simulink model "pwm_controlled_system"  (R2017a)
settings: Solver=FixedStepAuto  StartTime=0.0  StopTime=t_f  FixedStep=1e-6  RelTol=1e-3
values from neighbouring files (symbols this model uses):
  A = double(subs(A_sym, symbs, vals))    [load_params.m]
  B = double(subs(B_sym, symbs, vals))    [load_params.m]
  C = double(subs(C_sym, symbs, vals))    [load_params.m]    (also in load_pwm_avg_pred_controller.m = sysd.c; load_pwm_pred_controller.m = sysd.c)
  Ctilde = double(subs(Ctilde_sym, symbs, vals))    [load_params.m]
  torque_ref = n_val*k_i_val*i_ref    [load_params.m]
  Tpwm_val = 1e-2    (= 0.01)    [load_params.m]    (also in ss_value.m = 0.001)
  Ts_val = 1e-1    (= 0.1)    [load_params.m]    (also in ss_value.m = 0.011)
  Vcc_val = 12    [load_params.m]
  x0 = [0; 0]    [sim_controlled_system.m]
settings Model: Creator=brunolnetto  LastModifiedBy=brunolnetto

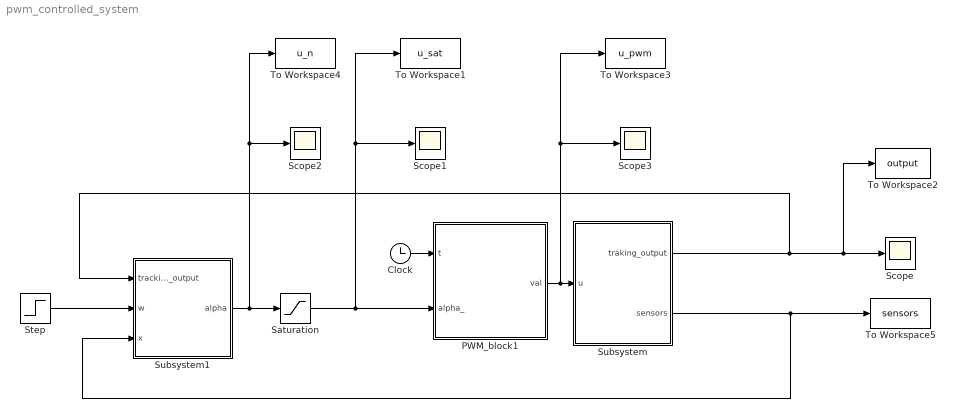
== system pwm_controlled_system ==
  Clock : Clock
  PWM_block1 : MATLAB Function  TreatAsAtomicUnit=on
  Saturation : Saturate  UpperLimit=1  LowerLimit=-1
  Scope{,1..3} (4 alike) : Scope
  Step : Step  Time=0  After=torque_ref  SampleTime=Ts_val
  Subsystem : Subsystem
  Subsystem1 : Subsystem
  To Workspace1 : ToWorkspace  VariableName=u_sat  SaveFormat=Structure With Time  SampleTime=-1
  To Workspace2 : ToWorkspace  VariableName=output  SaveFormat=Structure With Time  SampleTime=-1
  To Workspace3 : ToWorkspace  VariableName=u_pwm  SaveFormat=Structure With Time  SampleTime=-1
  To Workspace4 : ToWorkspace  VariableName=u_n  SaveFormat=Structure With Time  SampleTime=-1
  To Workspace5 : ToWorkspace  VariableName=sensors  SaveFormat=Structure With Time  SampleTime=-1
  wires:
  Subsystem/1(traking_output) -> To Workspace2/1, Scope/1, Subsystem1/1(tracking_output)
  Subsystem/2(sensors) -> To Workspace5/1, Subsystem1/3(x)
  Step/1 -> Subsystem1/2(w)
  Clock/1 -> PWM_block1/1(t)
  Subsystem1/1(alpha) -> To Workspace4/1, Scope2/1, Saturation/1
  Saturation/1 -> PWM_block1/2(alpha_), Scope1/1, To Workspace1/1
  PWM_block1/1(val) -> Scope3/1, To Workspace3/1, Subsystem/1(u)

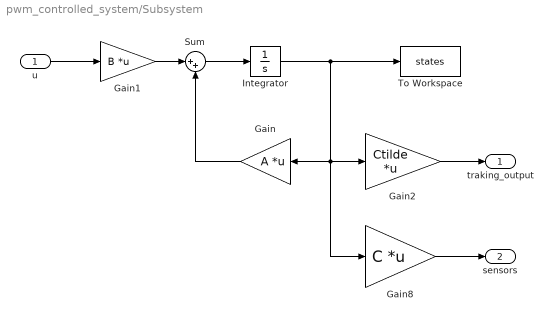
== system pwm_controlled_system/Subsystem ==
  u : Inport
  Gain : Gain  Gain=A  Multiplication=Matrix(K*u) (u vector)
  Gain1 : Gain  Gain=B  Multiplication=Matrix(K*u) (u vector)
  Gain2 : Gain  Gain=Ctilde  Multiplication=Matrix(K*u) (u vector)
  Gain8 : Gain  Gain=C  Multiplication=Matrix(K*u) (u vector)
  Integrator : Integrator  InitialCondition=x0
  Sum : Sum  Inputs=|++
  To Workspace : ToWorkspace  VariableName=states  SaveFormat=Structure With Time  SampleTime=-1
  traking_output : Outport
  sensors : Outport  Port=2
  wires:
  Gain8/1 -> sensors/1
  Gain1/1 -> Sum/1
  Integrator/1 -> To Workspace/1, Gain2/1, Gain8/1, Gain/1
  u/1 -> Gain1/1
  Gain/1 -> Sum/2
  Sum/1 -> Integrator/1
  Gain2/1 -> traking_output/1

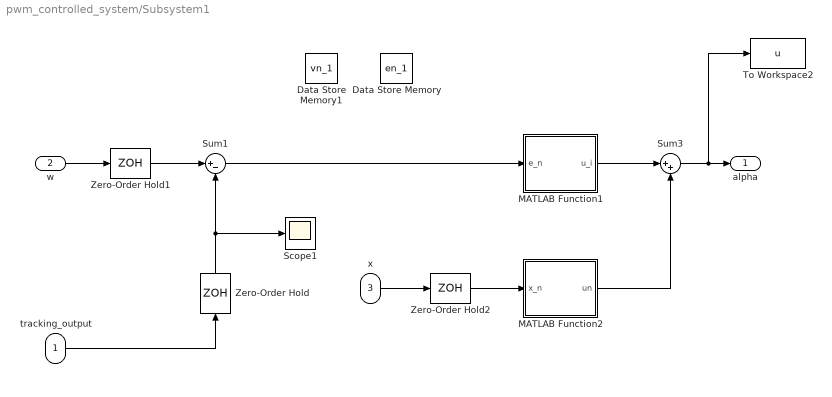
== system pwm_controlled_system/Subsystem1 ==
  tracking_output : Inport
  w : Inport  Port=2
  x : Inport  Port=3
  Data Store Memory : DataStoreMemory  DataStoreName=en_1  ReadBeforeWriteMsg=warning  WriteAfterWriteMsg=warning  WriteAfterReadMsg=warning  InitialValue=e0  ShowAdditionalParam=off  OutDataTypeStr=double
  Data Store Memory1 : DataStoreMemory  DataStoreName=vn_1  ReadBeforeWriteMsg=warning  WriteAfterWriteMsg=warning  WriteAfterReadMsg=warning  ShowAdditionalParam=off  OutDataTypeStr=double
  MATLAB Function1 : MATLAB Function  TreatAsAtomicUnit=on
  MATLAB Function2 : MATLAB Function  TreatAsAtomicUnit=on
  Scope1 : Scope
  Sum1 : Sum  Inputs=|+-
  Sum3 : Sum  Inputs=|++
  To Workspace2 : ToWorkspace  VariableName=u  SaveFormat=Structure With Time  SampleTime=-1
  Zero-Order Hold : ZeroOrderHold  SampleTime=Ts_val
  Zero-Order Hold1 : ZeroOrderHold  SampleTime=Ts_val
  Zero-Order Hold2 : ZeroOrderHold  SampleTime=Ts_val
  alpha : Outport
  wires:
  Zero-Order Hold1/1 -> Sum1/1
  MATLAB Function1/1(u_i) -> Sum3/1
  MATLAB Function2/1(un) -> Sum3/2
  tracking_output/1 -> Zero-Order Hold/1
  Zero-Order Hold2/1 -> MATLAB Function2/1(x_n)
  Sum3/1 -> To Workspace2/1, alpha/1
  x/1 -> Zero-Order Hold2/1
  Sum1/1 -> MATLAB Function1/1(e_n)
  Zero-Order Hold/1 -> Scope1/1, Sum1/2
  w/1 -> Zero-Order Hold1/1

== matlab function pwm_controlled_system/Subsystem1/MATLAB Function1 ==
  data: e_n input; u_i output; en_1 data_store_memory; vn_1 data_store_memory; params parameter
function u_i = integrator(e_n, params)
    global vn_1;
    global en_1;
    
    v_n = vn_1 + en_1 ;
    
    u_i = params.Ki * v_n;
    
    en_1 = e_n;
    vn_1 = v_n;
end

== matlab function pwm_controlled_system/Subsystem1/MATLAB Function2 ==
  data: x_n input; un output; en_1 data_store_memory; vn_1 data_store_memory; params parameter
function un = proportional(x_n, params)
    un = - params.Kp*x_n;
end

== matlab function pwm_controlled_system/PWM_block1 ==
  data: t input; alpha_ input; val output; Vcc_val parameter; Tpwm_val parameter
function val = pwm_signal(t, alpha_, Vcc_val, Tpwm_val)
    % Static variable
    persistent t0;
    
    if(isempty(t0))
        t0 = 0;
    end
        
    % PWM generation
    if(t == 0)
        t0 = 0;
    end
    
    if(t - t0 > Tpwm_val)
        t0 = t;
    end
    
    % Inner time interval
    t_i = t - t0;
    
    abs_alpha = abs(alpha_);
    sign_alpha = sign(alpha_);
    
    if(t_i <= abs_alpha*Tpwm_val)
        val = sign_alpha*Vcc_val;
    else
        val = 0;
    end
end
